simulink model "altitude_from_pitch_loop"  (R2019a)
settings: Solver=VariableStepAuto  StartTime=0.0  StopTime=10000  RelTol=1e-3
undefined symbols (not defined in the file or in its folder): AP, trans_func
settings Model: Creator=nikhil  LastModifiedBy=VTOL_HYD

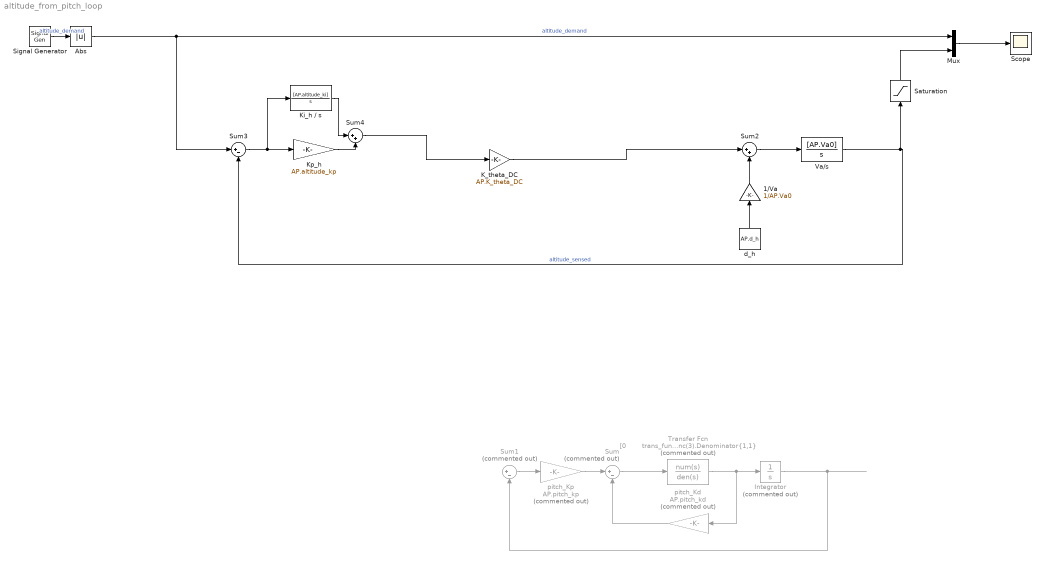
== system altitude_from_pitch_loop ==
  1/Va : Gain  Gain=1/AP.Va0
  Abs : Abs
  Integrator : Integrator  Commented=on
  K_theta_DC : Gain  Gain=AP.K_theta_DC
  Ki_h / s : TransferFcn  Numerator=[AP.altitude_ki]  Denominator=[1 0]
  Kp_h : Gain  Gain=AP.altitude_kp
  Mux : Mux  Inputs=2
  Saturation : Saturate  UpperLimit=10000
  Scope : Scope
  Signal Generator : SignalGenerator  WaveForm=sawtooth  Amplitude=100  Frequency=.02  Units=rad/sec
  Sum : Sum  Commented=on  Inputs=|+-
  Sum1 : Sum  Commented=on  Inputs=|+-
  Sum2 : Sum  Inputs=|++
  Sum3 : Sum  Inputs=|+-
  Sum4 : Sum  Inputs=|++
  Transfer Fcn : TransferFcn  Commented=on  Numerator="[0        trans_func(3).Numerator{1,1}(3)       0]"  Denominator=trans_func(3).Denominator{1,1}
  Va/s : TransferFcn  Numerator=[AP.Va0]  Denominator=[1 0]
  d_h : Constant  Value=AP.d_h
  pitch_Kd : Gain  Commented=on  Gain=AP.pitch_kd
  pitch_Kp : Gain  Commented=on  Gain=AP.pitch_kp
  wires:
  Va/s/1 -> Saturation/1, Sum3/2  "altitude_sensed"
  Mux/1 -> Scope/1
  Sum4/1 -> K_theta_DC/1
  Ki_h / s/1 -> Sum4/1
  Kp_h/1 -> Sum4/2
  Abs/1 -> Sum3/1, Mux/1  "altitude_demand"
  Sum3/1 -> Ki_h / s/1, Kp_h/1
  1/Va/1 -> Sum2/2
  d_h/1 -> 1/Va/1
  Sum2/1 -> Va/s/1
  Saturation/1 -> Mux/2
  Integrator/1 -> Sum1/2
  Sum/1 -> Transfer Fcn/1
  pitch_Kp/1 -> Sum/1
  pitch_Kd/1 -> Sum/2
  Sum1/1 -> pitch_Kp/1
  Transfer Fcn/1 -> pitch_Kd/1, Integrator/1
  K_theta_DC/1 -> Sum2/1
  Signal Generator/1 -> Abs/1  "altitude_demand"
